simulink model "drehzahlregelung_pi_regler_stoerung"  (R2025b)
settings: Solver=VariableStepAuto  StartTime=0.0  StopTime=10.0  RelTol=1e-3
values from neighbouring files (symbols this model uses):
  final_value_regler_pi = 300    [a3.m]    (also in params.m = 100)
  final_value_stoerung = 0.01    [params.m]
  init_value_regler_pi = 0    [params.m]
  init_value_stoerung = 0    [params.m]
  J = 0.4e9    (= 400000000)    [a1_params.m]    (also in params.m = 0.0004)
  K = 30e-3    (= 0.03)    [a1_params.m]    (also in params.m)
  Kr = 0.1    [params.m]
  L = 120e-6    (= 0.00012)    [a1_params.m]    (also in params.m)
  R = 6    [a1_params.m]    (also in params.m)
  sample_time_regler_pi = 0    [params.m]
  sample_time_stoerung = 0    [params.m]
  sat_max = 10    [params.m]
  sat_min = -10    [params.m]
  step_time_regler_pi = 1    [params.m]
  step_time_stoerung = 10    [params.m]
  Tn = 27    [params.m]
libraries: slpidlib x1
settings Model: Creator=rishabh  LastModifiedBy=rishabh

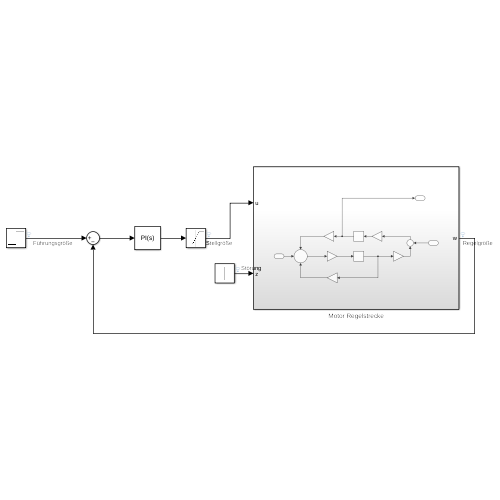
[thumbnail: Simulink's stored preview of the top-level diagram]
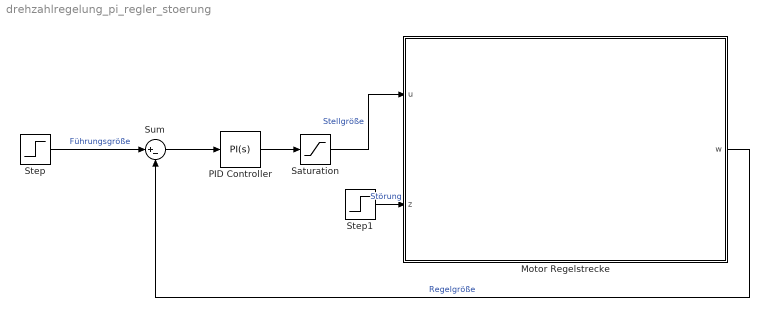
== system drehzahlregelung_pi_regler_stoerung ==
  Motor Regelstrecke : Subsystem
  PID Controller : slpidlib/PID Controller  Controller=PI  Form=Parallel  TimeDomain=Continuous-time  UseExternalTs=off  SampleTime=-1  IntegratorMethod=Forward Euler  FilterMethod=Forward Euler  ControllerParametersSource=internal  P=Kr  I=1/Tn  UseKiTs=off  D=0  UseExternalDerivativeSource=off  N=100  UseFilter=on  TunerSelectOption=Transfer Function Based (PID Tuner App)  InitialConditionSource=internal  InitialConditionForIntegrator=0  InitialConditionForFilter=0  DifferentiatorICPrevScaledInput=0  ExternalReset=none  TrackingMode=off  Kt=1  LimitOutput=off  SatLimitsSource=internal  UpperSaturationLimit=inf  LowerSaturationLimit=-inf  LinearizeAsGain=on  AntiWindupMode=none  Kb=1  LimitIntegrator=off  UpperIntegratorSaturationLimit=inf  LowerIntegratorSaturationLimit=-inf  POutMin=[]  POutMax=[]  IOutMin=[]  IOutMax=[]  DOutMin=[]  DOutMax=[]  NOutMin=[]  NOutMax=[]  SumOutMin=[]  SumOutMax=[]  SaturationOutMin=[]  SaturationOutMax=[]  PParamMin=[]  PParamMax=[]  IParamMin=[]  IParamMax=[]  DParamMin=[]  DParamMax=[]  NParamMin=[]  NParamMax=[]  KbParamMin=[]  KbParamMax=[]  KtParamMin=[]  KtParamMax=[]  KbOutMin=[]  KbOutMax=[]  KtOutMin=[]  KtOutMax=[]  IntegratorOutMin=[]  IntegratorOutMax=[]  FilterOutMin=[]  FilterOutMax=[]  SumI1OutMin=[]  SumI1OutMax=[]  SumI2OutMin=[]  SumI2OutMax=[]  SumI3OutMin=[]  SumI3OutMax=[]  SumI4OutMin=[]  SumI4OutMax=[]  SumDOutMin=[]  SumDOutMax=[]  DifferentiatorOutMin=[]  DifferentiatorOutMax=[]  FilterDiffOutCoefMin=[]  FilterDiffOutCoefMax=[]  ReciprocalOutMin=[]  ReciprocalOutMax=[]  SumDenOutMin=[]  SumDenOutMax=[]  SumNumOutMin=[]  SumNumOutMax=[]  DivideOutMin=[]  DivideOutMax=[]  UdiffTsProdOutMin=[]  UdiffTsProdOutMax=[]  NTsProdOutMin=[]  NTsProdOutMax=[]  UintegralTsProdOutMin=[]  UintegralTsProdOutMax=[]  UngainTsProdOutMin=[]  UngainTsProdOutMax=[]  ClampingZeroOutDataTypeStr=Inherit: Inherit via back propagation  ClampingZeroOutMin=[]  ClampingZeroOutMax=[]  FilterDenConstantOutDataTypeStr=Inherit: Inherit via back propagation  FilterDenConstantOutMin=[]  FilterDenConstantOutMax=[]  PCopyOutDataTypeStr=Inherit: Inherit via back propagation  PCopyOutMin=[]  PCopyOutMax=[]  NCopyOutDataTypeStr=Inherit: Inherit via back propagation  NCopyOutMin=[]  NCopyOutMax=[]  IntegratorContinuousStateAttributes=''  IntegratorStateMustResolveToSignalObject=off  IntegratorRTWStateStorageClass=Auto  FilterContinuousStateAttributes=''  FilterStateMustResolveToSignalObject=off  FilterRTWStateStorageClass=Auto  ParallelPVariant=InternalParameters  IdealPVariant=Disabled  IVariant=InternalParameters  DVariant=Disabled  IntegratorVariant=Continuous  SatVariant=Disabled  AWVariant=Passthrough  PCopyVariant=Disabled  TRVariant=Disabled  FdbkBlocksVariant=Forward  IdealPFdbkVariant=Disabled  SatFdbkVariant=Disabled  DerivativeFilterVariant=Disabled  NVariant=Disabled  NCopyVariant=Disabled_SignalSpec  FilterICVariant=Disabled  IntegratorICVariant=InternalICs  ExternalResetVariant=Disabled  TRSumVariant=Passthrough  SumFdbkVariant=Disabled  SumVariant=Sum_PI  TsampFilterVariant=InternalTs  TsampNgainVariant=Passthrough  TsampIntegralVariant=Disabled_SignalSpec  ExternalSaturationOutDataTypeStr=Inherit: Same as second input  DerivativeSourceVariant=Disabled  PreIntVariant=InternalPreInt
  Saturation : Saturate  UpperLimit=sat_max  LowerLimit=sat_min
  Step : Step  Time=step_time_regler_pi  Before=init_value_regler_pi  After=final_value_regler_pi  SampleTime=sample_time_regler_pi
  Step1 : Step  Time=step_time_stoerung  Before=init_value_stoerung  After=final_value_stoerung  SampleTime=sample_time_stoerung
  Sum : Sum  Inputs=|+-
  wires:
  Sum/1 -> PID Controller/1
  PID Controller/1 -> Saturation/1
  Saturation/1 -> Motor Regelstrecke/1(u)  "Stellgröße"
  Step/1 -> Sum/1  "Führungsgröße"
  Step1/1 -> Motor Regelstrecke/2(z)  "Störung"
  Motor Regelstrecke/1(w) -> Sum/2  "Regelgröße"

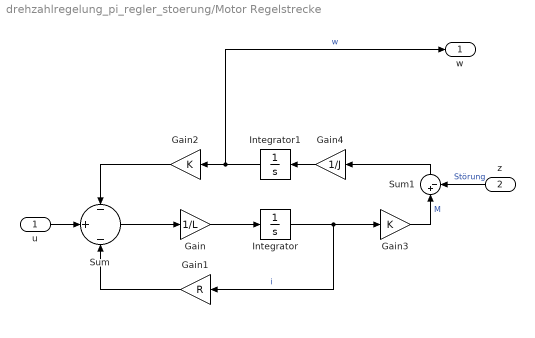
== system drehzahlregelung_pi_regler_stoerung/Motor Regelstrecke ==
  u : Inport
  z : Inport  Port=2
  Gain : Gain  Gain=1/L
  Gain1 : Gain  Gain=R
  Gain2 : Gain  Gain=K
  Gain3 : Gain  Gain=K
  Gain4 : Gain  Gain=1/J
  Integrator : Integrator
  Integrator1 : Integrator
  Sum : Sum  Inputs=-|+|-
  Sum1 : Sum  Inputs=|+-
  w : Outport
  wires:
  u/1 -> Sum/2
  Gain4/1 -> Integrator1/1
  Sum/1 -> Gain/1
  Integrator1/1 -> w/1, Gain2/1  "w"
  Gain2/1 -> Sum/1
  Gain3/1 -> Sum1/1  "M"
  Gain1/1 -> Sum/3
  Gain/1 -> Integrator/1
  Integrator/1 -> Gain1/1, Gain3/1  "i"
  z/1 -> Sum1/2  "Störung"
  Sum1/1 -> Gain4/1
